simulink model "Q2_3"  (R2024b)
settings: Solver=ode4  StartTime=0.0  StopTime=10  FixedStep=Ts  RelTol=1e-3
undefined symbols (not defined in the file): dspblkCoreblockFVToolHelper, G_r1_u2, G_r1_y1, G_r1_y3, G_r2_y2, G_r2_y3, gcbh, sys_d, Ts
settings Model: Creator=liou-  LastModifiedBy=liou-

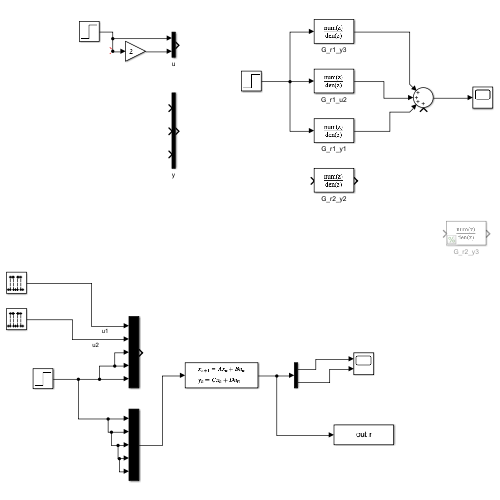
[thumbnail: Simulink's stored preview of the top-level diagram]
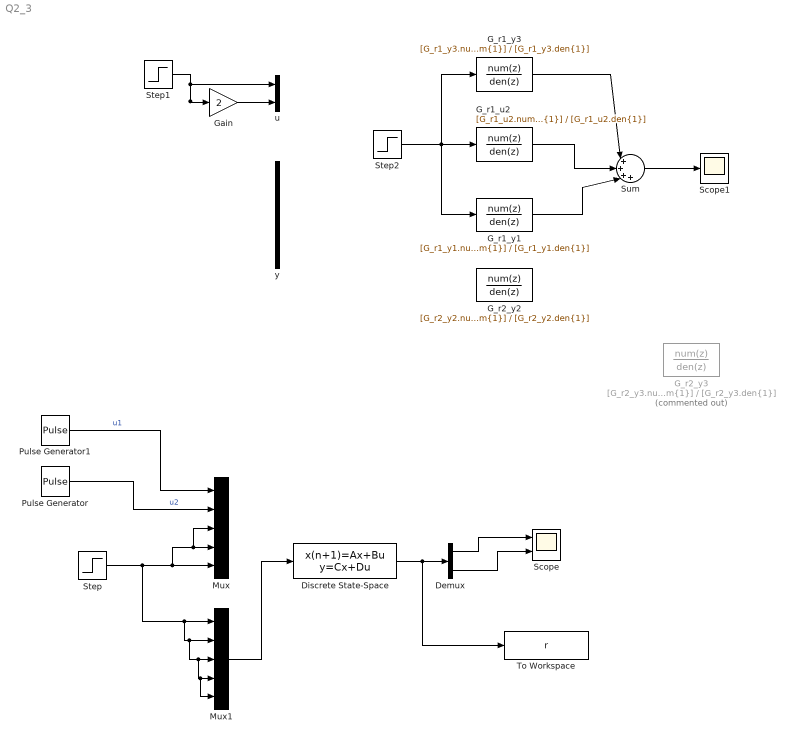
== system Q2_3 ==
  Demux : Demux  Outputs=2
  Discrete State-Space : DiscreteStateSpace  A=sys_d.A  B=sys_d.B  C=sys_d.C  D=sys_d.D  SampleTime=Ts
  G_r1_u2 : DiscreteTransferFcn  LoadFcn=dspblkCoreblockFVToolHelper(gcbh,'load');  Numerator=[G_r1_u2.num{1}]  Denominator=[G_r1_u2.den{1}]
      settings: CopyFcn=dspblkCoreblockFVToolHelper(gcbh,'copy');  DeleteFcn=dspblkCoreblockFVToolHelper(gcbh,'close');  ModelCloseFcn=dspblkCoreblockFVToolHelper(gcbh,'close');  PreSaveFcn=dspblkCoreblockFVToolHelper(gcbh,'presave');  PostSaveFcn=dspblkCoreblockFVToolHelper(gcbh,'postsave');  CloseFcn=dspblkCoreblockFVToolHelper(gcbh,'close');
  G_r1_y1 : DiscreteTransferFcn  LoadFcn=dspblkCoreblockFVToolHelper(gcbh,'load');  Numerator=[G_r1_y1.num{1}]  Denominator=[G_r1_y1.den{1}]
      settings: CopyFcn=dspblkCoreblockFVToolHelper(gcbh,'copy');  DeleteFcn=dspblkCoreblockFVToolHelper(gcbh,'close');  ModelCloseFcn=dspblkCoreblockFVToolHelper(gcbh,'close');  PreSaveFcn=dspblkCoreblockFVToolHelper(gcbh,'presave');  PostSaveFcn=dspblkCoreblockFVToolHelper(gcbh,'postsave');  CloseFcn=dspblkCoreblockFVToolHelper(gcbh,'close');
  G_r1_y3 : DiscreteTransferFcn  LoadFcn=dspblkCoreblockFVToolHelper(gcbh,'load');  Numerator=[G_r1_y3.num{1}]  Denominator=[G_r1_y3.den{1}]
      settings: CopyFcn=dspblkCoreblockFVToolHelper(gcbh,'copy');  DeleteFcn=dspblkCoreblockFVToolHelper(gcbh,'close');  ModelCloseFcn=dspblkCoreblockFVToolHelper(gcbh,'close');  PreSaveFcn=dspblkCoreblockFVToolHelper(gcbh,'presave');  PostSaveFcn=dspblkCoreblockFVToolHelper(gcbh,'postsave');  CloseFcn=dspblkCoreblockFVToolHelper(gcbh,'close');
  G_r2_y2 : DiscreteTransferFcn  LoadFcn=dspblkCoreblockFVToolHelper(gcbh,'load');  Numerator=[G_r2_y2.num{1}]  Denominator=[G_r2_y2.den{1}]
      settings: CopyFcn=dspblkCoreblockFVToolHelper(gcbh,'copy');  DeleteFcn=dspblkCoreblockFVToolHelper(gcbh,'close');  ModelCloseFcn=dspblkCoreblockFVToolHelper(gcbh,'close');  PreSaveFcn=dspblkCoreblockFVToolHelper(gcbh,'presave');  PostSaveFcn=dspblkCoreblockFVToolHelper(gcbh,'postsave');  CloseFcn=dspblkCoreblockFVToolHelper(gcbh,'close');
  G_r2_y3 : DiscreteTransferFcn  Commented=on  LoadFcn=dspblkCoreblockFVToolHelper(gcbh,'load');  Numerator=[G_r2_y3.num{1}]  Denominator=[G_r2_y3.den{1}]
      settings: CopyFcn=dspblkCoreblockFVToolHelper(gcbh,'copy');  DeleteFcn=dspblkCoreblockFVToolHelper(gcbh,'close');  ModelCloseFcn=dspblkCoreblockFVToolHelper(gcbh,'close');  PreSaveFcn=dspblkCoreblockFVToolHelper(gcbh,'presave');  PostSaveFcn=dspblkCoreblockFVToolHelper(gcbh,'postsave');  CloseFcn=dspblkCoreblockFVToolHelper(gcbh,'close');
  Gain : Gain  Gain=2
  Mux : Mux  Inputs=5
  Mux1 : Mux  Inputs=5
  Pulse Generator : DiscretePulseGenerator  Period=20  PulseWidth=5
  Pulse Generator1 : DiscretePulseGenerator  Period=8  PulseWidth=5
  Scope : Scope  NumInputPorts=2
  Scope1 : Scope
  Step : Step  SampleTime=0
  Step1 : Step  SampleTime=0
  Step2 : Step  SampleTime=0
  Sum : Sum  Inputs=|++++
  To Workspace : ToWorkspace  VariableName=r  SaveFormat=Timeseries  SampleTime=-1
  u : Mux  Inputs=2
  y : Mux  Inputs=3
  wires:
  Pulse Generator1/1 -> Mux/1  "u1"
  Pulse Generator/1 -> Mux/2  "u2"
  Step/1 -> Mux1/5, Mux1/4, Mux1/3, Mux1/2, Mux1/1, Mux/3, Mux/4, Mux/5
  Discrete State-Space/1 -> To Workspace/1, Demux/1
  Demux/1 -> Scope/1
  Demux/2 -> Scope/2
  Mux1/1 -> Discrete State-Space/1
  G_r1_y1/1 -> Sum/3
  G_r1_u2/1 -> Sum/2
  G_r1_y3/1 -> Sum/1
  Sum/1 -> Scope1/1
  Step1/1 -> u/1, Gain/1
  Gain/1 -> u/2
  Step2/1 -> G_r1_y1/1, G_r1_y3/1, G_r1_u2/1
